simulink model "Voltage_measurement_Above"  (R2021b)
settings: Solver=FixedStepAuto  StartTime=0.0  StopTime=inf  FixedStep=0.01  RelTol=1e-3  EnableMultiTasking=on
libraries: arduinolib x1
settings Model: ExtModeTrigDuration=2  Creator=bouss  LastModifiedBy=bouss
settings DataIOCC: ReturnWorkspaceOutputs=off
settings OptimizationCC: EnhancedBackFolding=on  PassReuseOutputArgsAs=Individual arguments  ZeroExternalMemoryAtStartup=off  ZeroInternalMemoryAtStartup=off  MaxStackSize=64  OptimizeBlockOrder=speed  DifferentSizesBufferReuse=on  OptimizationCustomize=off  EfficientTunableParamExpr=on
settings DebuggingCC: ParameterTunabilityLossMsg=error
settings HardwareCC: ProdBitPerInt=16  ProdBitPerPointer=16  ProdBitPerSizeT=16  ProdBitPerPtrDiffT=16  ProdLargestAtomicFloat=None  ProdWordSize=8  ProdHWDeviceType=Atmel->AVR
settings SFSimCC: MATLABDynamicMemAlloc=off
settings RTWCC: Description=Embedded Coder  SystemTargetFile=ert.tlc  HardwareBoard=Arduino Uno  TemplateMakefile=ert_default_tmf  Toolchain=Arduino AVR  BuildConfiguration=Faster Runs
settings CodeAppCC: ForceParamTrailComments=on  IgnoreCustomStorageClasses=off  OperatorAnnotations=on  SimulinkDataObjDesc=on  SFDataObjDesc=on  InsertBlockDesc=on
settings ERTTargetCC: SupportContinuousTime=on  SupportVariableSizeSignals=on  ExtModeTransport=3  ExtModeStaticAlloc=on  ExtModeStaticAllocSize=250  ExtModeMexFile=ext_xcp  ExtModeIntrfLevel=Level2 - Open

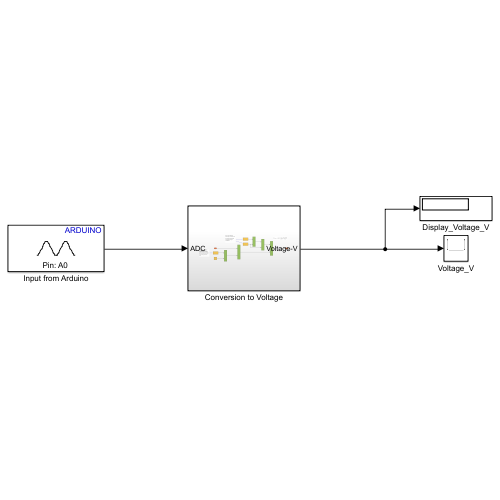
[thumbnail: Simulink's stored preview of the top-level diagram]
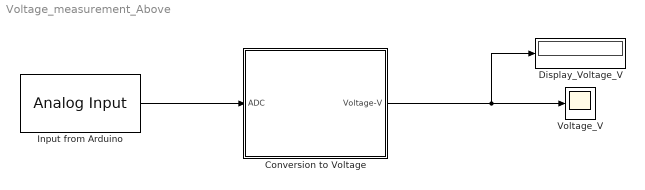
== system Voltage_measurement_Above ==
  Conversion to Voltage : Subsystem
  Display_Voltage_V : Display
  Input from Arduino : arduinolib/Analog Input  pinNumber=0  ReadResultsOnly=off  ConversionTriggerSource=Software  ExternalTriggerType=uint32( 0 )  OutputDataType=uint16  EnableConversionCompleteNotify=off  EnableOuputStatus=off  SampleTime=0.01  blockPlatform=arduino
  Voltage_V : Scope
  wires:
  Conversion to Voltage/1(Voltage-V) -> Display_Voltage_V/1, Voltage_V/1
  Input from Arduino/1 -> Conversion to Voltage/1(ADC)

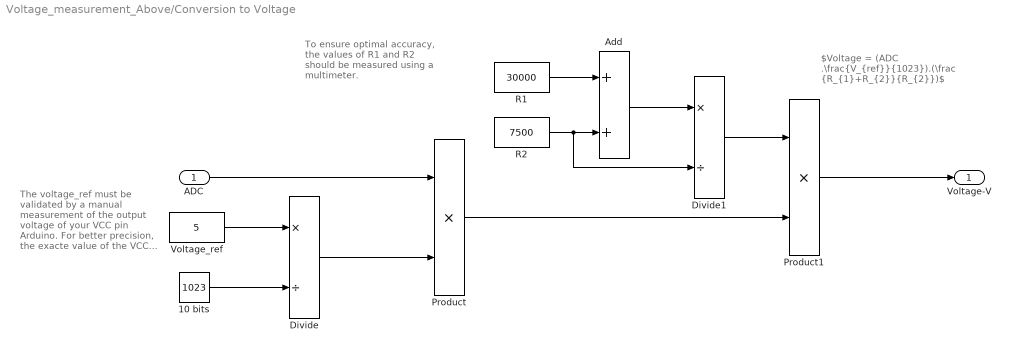
== system Voltage_measurement_Above/Conversion to Voltage ==
  note: $Voltage = (ADC .\frac{V_{ref}}{1023}).(\frac {R_{1}+R_{2}}{R_{2}})$
  note: The voltage_ref must be validated by a manual measurement of the output voltage of your VCC pin Arduino. For better precision, the exacte value of the VCC output voltage should be used.
  note: To ensure optimal accuracy, the values of R1 and R2 should be measured using a multimeter.
  ADC : Inport
  10 bits : Constant  Value=1023
  Add : Sum
  Divide : Product  Inputs=*/
  Divide1 : Product  Inputs=*/
  Product : Product
  Product1 : Product
  R1 : Constant  Value=30000
  R2 : Constant  Value=7500
  Voltage_ref : Constant  Value=5
  Voltage-V : Outport
  wires:
  Voltage_ref/1 -> Divide/1
  10 bits/1 -> Divide/2
  Divide/1 -> Product/2
  ADC/1 -> Product/1
  R1/1 -> Add/1
  R2/1 -> Divide1/2, Add/2
  Add/1 -> Divide1/1
  Divide1/1 -> Product1/1
  Product/1 -> Product1/2
  Product1/1 -> Voltage-V/1
